simulink model "Anti_Wind_up"  (R2020a)
settings: Solver=VariableStepAuto  StartTime=0.0  StopTime=20.0  RelTol=1e-3
libraries: simulink x1
settings Model: Creator=Emil  LastModifiedBy=Emil

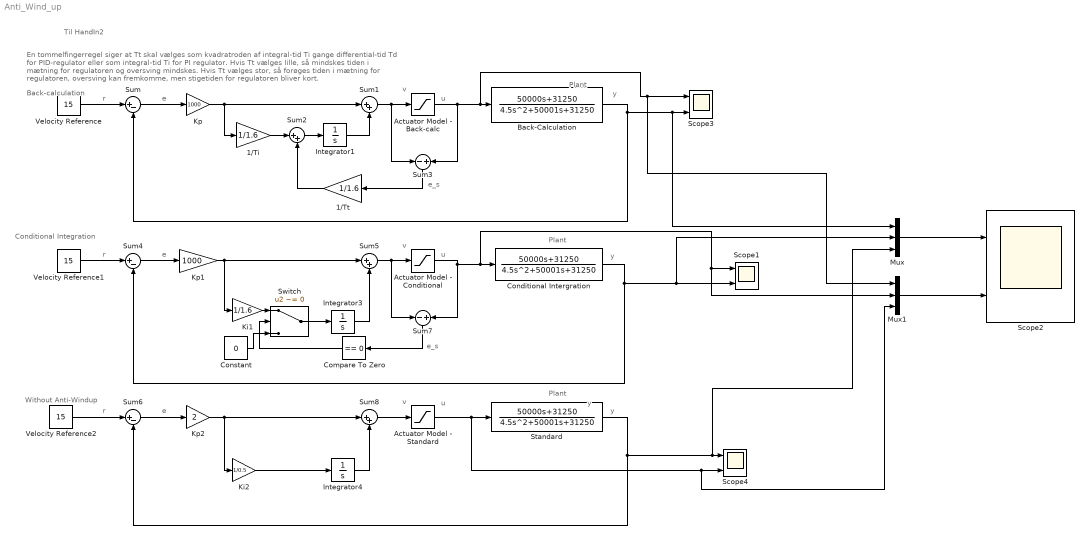
== system Anti_Wind_up ==
  note: Til HandIn2
  note: u
  note: v
  note: r
  note: e_s
  note: e
  note: r
  note: r
  note: e
  note: En tommelfingerregel siger at Tt skal vælges som kvadratroden af integral-tid Ti gange differential-tid Td for PID-regulator eller som integral-tid Ti for PI regulator.
      | Hvis Tt vælges lille, så mindskes tiden i mætning for regulatoren og oversving mindskes. Hvis Tt vælges stor, så forøges tiden i mætning for regulatoren, oversving kan fremkomme, men stigetiden for regulatoren bliver kort.
  note: Plant
  note: y
  note: e
  note: y
  note: v
  note: Without Anti-Windup
  note: e_s
  note: Back-calculation
  note: u
  note: Conditional Integration
  note: Plant
  note: y
  note: Plant
  note: v
  note: u
  note: y
  1/Ti : Gain  Gain=1/1.6
  1/Tt : Gain  Gain=1/1.6
  Actuator Model - Back-calc : Saturate  UpperLimit=3000  LowerLimit=-3000
  Actuator Model - Conditional : Saturate  UpperLimit=3000  LowerLimit=-3000
  Actuator Model - Standard : Saturate  UpperLimit=3000  LowerLimit=-3000
  Back-Calculation : TransferFcn  Numerator=[50000 31250]  Denominator=[4.5 50001 31250]
  Compare To Zero : simulink/Logic and Bit Operations/Compare To Zero  relop===  OutDataTypeStr=boolean
  Conditional Intergration : TransferFcn  Numerator=[50000 31250]  Denominator=[4.5 50001 31250]
  Constant : Constant  Value=0
  Integrator1 : Integrator
  Integrator3 : Integrator
  Integrator4 : Integrator
  Ki1 : Gain  Gain=1/1.6
  Ki2 : Gain  Gain=1/0.5
  Kp : Gain  Gain=1000
  Kp1 : Gain  Gain=1000
  Kp2 : Gain  Gain=2
  Mux : Mux  Inputs=3
  Mux1 : Mux  Inputs=3
  Scope{1..4} (4 alike) : Scope  NumInputPorts=2
  Standard : TransferFcn  Numerator=[50000 31250]  Denominator=[4.5 50001 31250]
  Sum : Sum  Inputs=|+-
  Sum{1..2,5,8} (4 alike) : Sum  Inputs=|++
  Sum3 : Sum  Inputs=-+
  Sum4 : Sum  Inputs=|+-
  Sum6 : Sum  Inputs=|+-
  Sum7 : Sum  Inputs=-+
  Switch : Switch  Criteria=u2 ~= 0
  Velocity Reference : Constant  Value=15
  Velocity Reference1 : Constant  Value=15
  Velocity Reference2 : Constant  Value=15
  wires:
  Sum4/1 -> Kp1/1
  Sum/1 -> Kp/1
  Sum3/1 -> 1/Tt/1
  Actuator Model - Back-calc/1 -> Sum3/2, Scope3/1, Mux1/1, Back-Calculation/1
  1/Tt/1 -> Sum2/2
  Kp/1 -> 1/Ti/1, Sum1/1
  Sum8/1 -> Actuator Model - Standard/1
  Mux/1 -> Scope2/1
  Compare To Zero/1 -> Switch/2
  Sum5/1 -> Sum7/1, Actuator Model - Conditional/1
  Mux1/1 -> Scope2/2
  Standard/1 -> Mux/3, Scope4/1, Sum6/2
  1/Ti/1 -> Sum2/1
  Actuator Model - Conditional/1 -> Sum7/2, Conditional Intergration/1, Mux1/2, Scope1/1
  Ki2/1 -> Integrator4/1
  Integrator3/1 -> Sum5/2
  Ki1/1 -> Switch/1
  Integrator1/1 -> Sum1/2
  Kp2/1 -> Ki2/1, Sum8/1
  Back-Calculation/1 -> Sum/2, Mux/1, Scope3/2
  Actuator Model - Standard/1 -> Scope4/2, Mux1/3, Standard/1
  Sum2/1 -> Integrator1/1
  Sum1/1 -> Sum3/1, Actuator Model - Back-calc/1
  Integrator4/1 -> Sum8/2
  Velocity Reference2/1 -> Sum6/1
  Sum6/1 -> Kp2/1
  Constant/1 -> Switch/3
  Sum7/1 -> Compare To Zero/1
  Velocity Reference1/1 -> Sum4/1
  Conditional Intergration/1 -> Scope1/2, Mux/2, Sum4/2
  Velocity Reference/1 -> Sum/1
  Kp1/1 -> Sum5/1, Ki1/1
  Switch/1 -> Integrator3/1
